simulink model "ComponentPCtest"  (R2014b)
settings: Solver=FixedStepDiscrete  StartTime=0.0  StopTime=30  FixedStep=1  RelTol=1e-3
InitFcn:
  | clearAll;
  | 
  | 
  | p = PulseArray();
  | p.addPulse(Pulse([]));
  | 
  | % Vector of input pulse timings
  | num_pulses_start = 100;
  | timings = 0:13e-9:(num_pulses_start-1)*13e-9;
  | 
  | % Pulse sequence creation
  | inputsignal = zeros(length(timings)+100,1);
  | 
  | for i = 1:length(timings)
  |     pulse1 = Pulse([timings(i)]);
  |     %pulse2 = Pulse([timings(i)]);
  |     pA = PulseArray();
  |     pA.addPulse(pulse1);
  |     %pA.addPulse(pulse2);
  | 
  |     inputsignal(i) = pA.ID;
  | end
libraries: dspsrcs4 x1
settings Model: Creator=kunalmenda  LastModifiedBy=kunalmenda

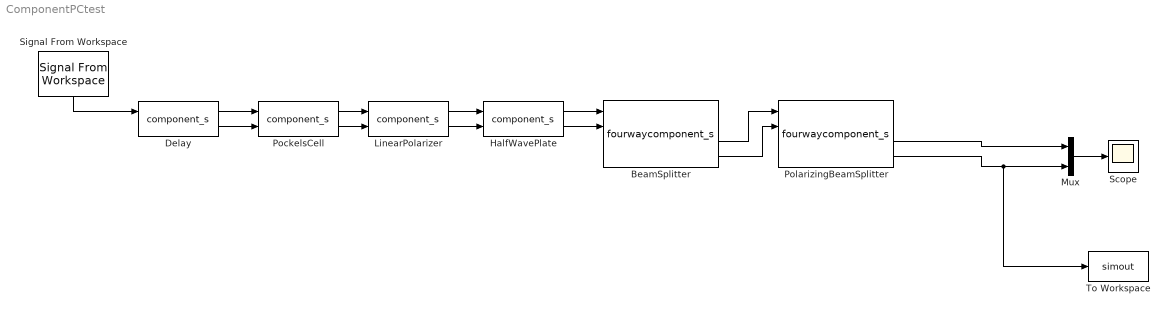
== system ComponentPCtest ==
  BeamSplitter : M-S-Function  FunctionName=fourwaycomponent_s  Parameters='BeamSplitter',Params  mask{Transmittance=0.50, Reflectance=0.50, Ghost=0.01}
      mask init:
      | Params.Transmittance = Transmittance;
      | Params.Reflectance = Reflectance;
      | Params.Ghost = Ghost;
      mask Display:
      | port_label('input',1,'TopIn');
      | port_label('input',2,'LeftIn');
      | port_label('input',3,'RightIn');
      | port_label('input',4,'BottomIn');
      | port_label('output',1,'TopOut');
      | port_label('output',2,'LeftOut');
      | port_label('output',3,'RightOut');
      | port_label('output',4,'BottomOut');
  Delay : M-S-Function  FunctionName=component_s  Parameters='Delay',Params  mask{DelayAmt=10e-9}
      mask prompts: DelayAmt "Delay Amout"
      mask init:
      | Params.DelayAmt = DelayAmt;
      mask Display:
      | port_label('input',1,'LeftIn');
      | port_label('input',2,'RightIn');
      | port_label('output',1,'LeftOut');
      | port_label('output',2,'RightOut');
  HalfWavePlate : M-S-Function  FunctionName=component_s  Parameters='HalfWavePlate',Params  mask{Psi=pi/4, Transmittence=0.99}
      mask init:
      | Params.Psi = Psi;
      | Params.Transmittence = Transmittence;
      mask Display:
      | port_label('input',1,'LeftIn');
      | port_label('input',2,'RightIn');
      | port_label('output',1,'LeftOut');
      | port_label('output',2,'RightOut');
  LinearPolarizer : M-S-Function  FunctionName=component_s  Parameters='LinearPolarizer',Params  mask{Psi=pi/4, Transmittence=0.81, ExtinctionRatio=200000000}
      mask init:
      | Params.Psi = Psi;
      | Params.Transmittence = Transmittence;
      | Params.ExtinctionRatio = ExtinctionRatio;
      mask Display:
      | port_label('input',1,'LeftIn');
      | port_label('input',2,'RightIn');
      | port_label('output',1,'LeftOut');
      | port_label('output',2,'RightOut');
  Mux : Mux  Inputs=2
  PockelsCell : M-S-Function  FunctionName=component_s  Parameters='PockelsCell',Params  mask{PCTimings=[-1,1,38,40,103,105,168,170,220,274]*1e-9, ControlPowers=[0.5000, 1.0000,1.0000, 1.0000, 0.5000], Psi=pi/4}
      mask prompts: PCTimings "PC Timings"; ControlPowers "Control Powers"
      mask init:
      | Params.PCTimings = PCTimings;
      | Params.ControlPowers = ControlPowers;
      | Params.Psi = Psi;
      mask Display:
      | port_label('input',1,'LeftIn');
      | port_label('input',2,'RightIn');
      | port_label('output',1,'LeftOut');
      | port_label('output',2,'RightOut');
  PolarizingBeamSplitter : M-S-Function  FunctionName=fourwaycomponent_s  Parameters='PolarizingBeamSplitter',Params  mask{Psi=pi/2, Transmittance=0.50, Reflectance=0.50, Ghost=0.01}
      mask init:
      | Params.Psi = Psi;
      | Params.Transmittance = Transmittance;
      | Params.Reflectance = Reflectance;
      | Params.Ghost = Ghost;
      mask Display:
      | port_label('input',1,'TopIn');
      | port_label('input',2,'LeftIn');
      | port_label('input',3,'RightIn');
      | port_label('input',4,'BottomIn');
      | port_label('output',1,'TopOut');
      | port_label('output',2,'LeftOut');
      | port_label('output',3,'RightOut');
      | port_label('output',4,'BottomOut');
  Scope : Scope
  Signal From Workspace : dspsrcs4/Signal From Workspace  X=inputsignal  Ts=1  nsamps=1  OutputAfterFinalValue=Setting to zero  ignoreOrWarnInputAndFrameLengths=off
  To Workspace : ToWorkspace  VariableName=simout  SaveFormat=Timeseries  SampleTime=-1
  wires:
  Mux/1 -> Scope/1
  Signal From Workspace/1 -> Delay/1
  Delay/1 -> PockelsCell/1
  Delay/2 -> PockelsCell/2
  PockelsCell/1 -> LinearPolarizer/1
  PockelsCell/2 -> LinearPolarizer/2
  LinearPolarizer/1 -> HalfWavePlate/1
  LinearPolarizer/2 -> HalfWavePlate/2
  HalfWavePlate/1 -> BeamSplitter/1
  HalfWavePlate/2 -> BeamSplitter/2
  BeamSplitter/3 -> PolarizingBeamSplitter/1
  BeamSplitter/4 -> PolarizingBeamSplitter/2
  PolarizingBeamSplitter/3 -> Mux/1
  PolarizingBeamSplitter/4 -> To Workspace/1, Mux/2
